simulink model "martins_version_wconv"  (R2023b)
settings: Solver=VariableStepAuto  StartTime=0.0  StopTime=Tend  RelTol=1e-3
undefined symbols (not defined in the file): C_dc, c_f, C_hv_km, Cagg, DiscIntNeverNeededParam, H_vsm, Ibase_hv, Ibase_lv, Ibase_mv, k_AD, k_d_vsm, k_decouple, k_ffv, k_ic, k_idc, k_mod, k_p_p_vsm, k_p_q_vsm, k_pc, k_pdc, k_vc, KG_LL, ki, KI_LL, ki_q, kp, KP_LL, kslope_VSC, L_comp, l_f, l_f_si1, l_grid, L_hv_km, l_t_ehvhv, l_t_hvmv, l_t_mvlv, L_Virt, Lagg, Lbase1v, length_export, omega_nom, P_aero_0, phase_shift_test_state, phase_shifts, pie_export, r_f, r_f_si1, r_grid, R_hv_km, r_t_ehvhv, r_t_hvmv, r_t_mvlv, R_Virt, Ragg, rocof_slope, Rocof_test_state, Sbase1, Tchange_gfm_ref, Tdelay, Trocof_end ... (+13)
libraries: slpidlib x11, spsFirstOrderFilterLib x3, cstblocks x1, simulink x1, spsSampleandHoldLib x1, spspowerguiLib x1
(part 2 of 3)

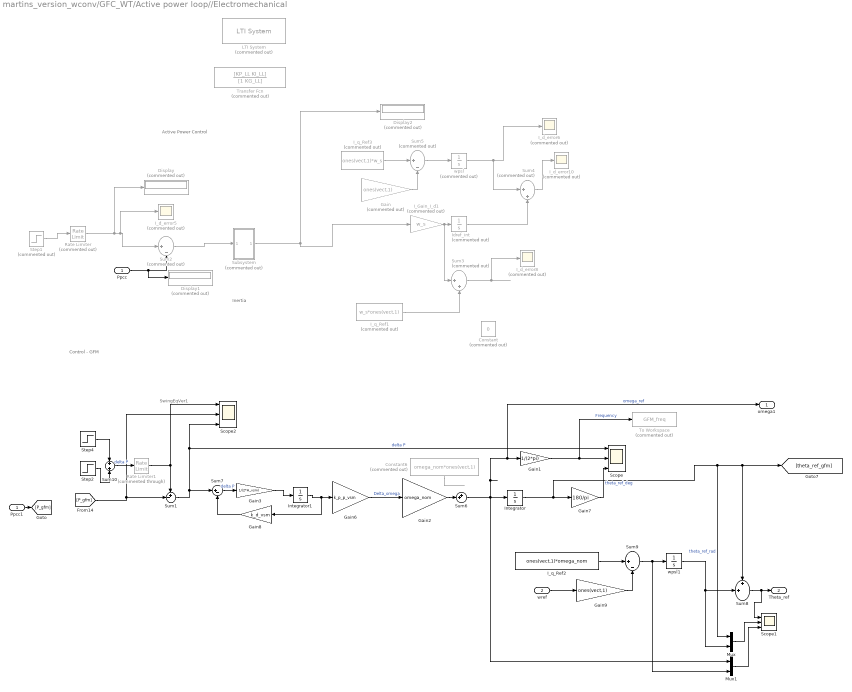
== system martins_version_wconv/GFC_WT/Active power loop//Electromechanical ==
  note: SwingEqVer1
  note: Active Power Control
  note: Inertia
  note: Control - GFM
  Ppcc : Inport  PortDimensions=vect
  wref : Inport  Port=2
  Constant : Constant  Commented=on  Value=0
  Constant6 : Constant  Commented=on  Value=omega_nom*ones(vect,1)
  Display : Display  Commented=on
  Display1 : Display  Commented=on
  Display2 : Display  Commented=on
  Gain : Gain  Commented=on  Gain=ones(vect,1)
  Gain1 : Gain  Gain=1/(2*pi)
  Gain2 : Gain  Gain=omega_nom
  Gain3 : Gain  Gain=1/(2*H_vsm)
  Gain6 : Gain  Gain=k_p_p_vsm
  Gain7 : Gain  Gain=180/pi
  Gain8 : Gain  Gain=k_d_vsm
  Gain9 : Gain  Gain=ones(vect,1)
  I_Gain_I_d1 : Gain  Commented=on  Gain=w_s
  I_d_error{5..6,8,10} (4 alike) : Scope  Commented=on
  I_q_Ref1 : Constant  Commented=on  Value=w_s*ones(vect,1)  SampleTime=-1
  I_q_Ref2 : Constant  Value=ones(vect,1)*omega_nom  SampleTime=-1
  I_q_Ref3 : Constant  Commented=on  Value=ones(vect,1)*w_s  SampleTime=-1
  "Idref_int " : Integrator  Commented=on  UpperSaturationLimit=300  LowerSaturationLimit=-100
  Integrator : Integrator  WrappedStateUpperValue=2*pi  WrappedStateLowerValue=0
  Integrator1 : Integrator
  LTI System : cstblocks/LTI System  Commented=on  sys=sys_mech  IC=[]  PadeOrder=0
  Mux : Mux  Inputs=2
  Mux1 : Mux  Inputs=2
  Ppcc1 : InportShadow  PortDimensions=vect
  Rate Limiter : RateLimiter  Commented=on  RisingSlewLimit=0.5  FallingSlewLimit=-0.5  SampleTimeMode=inherited
  Rate Limiter1 : RateLimiter  Commented=through  RisingSlewLimit=0.5  FallingSlewLimit=-0.5  SampleTimeMode=inherited
  Scope : Scope  NumInputPorts=3
  Scope1 : Scope  NumInputPorts=3
  Scope2 : Scope  NumInputPorts=3
  Step1 : Step  Commented=on  Time=2  Before=ones(vect,1)*0  After=ones(vect,1)*0.9  SampleTime=0
  Step2 : Step  Time=20  Before=0.0*ones(vect,1)  After=1*ones(vect,1)  SampleTime=Ts_power
  Step4 : Step  Time=8  Before=0.0*ones(vect,1)  After=P_aero_0*ones(vect,1)  SampleTime=Ts_power
  Subsystem : Subsystem  Commented=on
  Sum1 : Sum  Inputs=+-|
  Sum10 : Sum
  Sum2 : Sum  Commented=on  Inputs=|+-
  Sum3 : Sum  Commented=on  Inputs=|++
  Sum4 : Sum  Commented=on  Inputs=|++
  Sum5 : Sum  Commented=on  Inputs=|+-
  Sum6 : Sum  Inputs=++|
  Sum7 : Sum  Inputs=|+-
  Sum8 : Sum  Inputs=++|
  Sum9 : Sum  Inputs=|+-
  To Workspace : ToWorkspace  Commented=on  VariableName=GFM_freq  SaveFormat=Structure With Time  SampleTime=-1
  Transfer Fcn : TransferFcn  Commented=on  Numerator=[KP_LL KI_LL]  Denominator=[1 KG_LL]
  wpsl : Integrator  Commented=on  UpperSaturationLimit=300  LowerSaturationLimit=-100
  wpsl1 : Integrator  UpperSaturationLimit=300  LowerSaturationLimit=-100
  omega1 : Outport
  Theta_ref : Outport  Port=2
  wires:
  Ppcc/1 -> Sum2/2, Display1/1
  Subsystem/1(Out1) -> I_Gain_I_d1/1, Display2/1
  Sum4/1 -> I_d_error10/1
  I_Gain_I_d1/1 -> "Idref_int "/1, Sum3/1
  I_q_Ref3/1 -> Sum5/1
  ? -> Gain/1
  Sum5/1 -> wpsl/1
  wpsl/1 -> I_d_error6/1, Sum4/1
  I_q_Ref1/1 -> Sum3/2
  Sum3/1 -> I_d_error8/1
  "Idref_int "/1 -> Sum4/2
  Rate Limiter/1 -> I_d_error5/1, Sum2/1, Display/1
  Sum2/1 -> Subsystem/1(In1)
  Step1/1 -> Rate Limiter/1
  Gain/1 -> Sum5/2
  Step4/1 -> Sum10/1
  Ppcc1/1 -> [P_gfm]
  Gain1/1 -> To Workspace/1, Scope/2  "Frequency"
  Gain2/1 -> Sum6/2
  Constant6/1 -> ?
  Rate Limiter1/1 -> Scope2/1, Sum1/1
  Gain7/1 -> Scope/3  "theta_ref_deg"
  Gain6/1 -> Gain2/1  "Delta_omega"
  Sum6/1 -> Mux1/1, omega1/1, Gain1/1, Integrator/1  "omega_ref"
  Integrator/1 -> Mux/1, Sum8/1, [theta_ref_gfm], Gain7/1  "theta_ref_rad"
  Sum1/1 -> Scope/1, Scope2/3, Sum7/1  "delta P"
  Gain3/1 -> Integrator1/1
  Sum7/1 -> Gain3/1  "delta P"
  Gain8/1 -> Sum7/2
  Integrator1/1 -> Gain6/1, Gain8/1
  wref/1 -> Gain9/1
  wpsl1/1 -> Mux/2, Sum8/2
  I_q_Ref2/1 -> Sum9/1
  Gain9/1 -> Sum9/2
  Sum9/1 -> Mux1/2, wpsl1/1
  Sum8/1 -> Scope1/1, Theta_ref/1
  Mux/1 -> Scope1/2
  Mux1/1 -> Scope1/3
  [P_gfm] -> Sum1/2, Scope2/2
  Sum10/1 -> Rate Limiter1/1  "delta P"
  Step2/1 -> Sum10/2

== system martins_version_wconv/GFC_WT/Current Limit Logic1 ==
  note: Circular Current limiter
  I_ref_unsat : Inport
  Abs1 : Abs
  Constant3 : Constant
  Constant4 : Constant  Value=1.2
  Demux6 : Demux  Outputs=2
  Demux7 : Demux  Outputs=[vect vect]
  Display3 : Display
  Divide : Product  Inputs=*/
  Divide1 : Product  Inputs=*/
  First-Order Filter1 : spsFirstOrderFilterLib/First-Order Filter  FilterType=Lowpass  Tc=0.002  Ts=0  Initialize=on  Vac_Init=[0, 0, 60]  Vdc_Init=0  PlotResponse=off  FreqRange="[0,  200,  1]"
  GreaterThan1 : RelationalOperator  Operator=>  OutDataTypeStr=boolean  RndMeth=Simplest  InputSameDT=off
  I_d_error2 : Scope  Commented=on
  I_d_error3 : Scope  Commented=on
  I_d_error5 : Scope  Commented=on
  Kip12 : Gain
  Kip13 : Gain  Gain=1/1.2
  Mux6 : Mux  Inputs=[vect vect]
  Real-Imag to Complex1 : RealImagToComplex
  Switch1 : Switch  Threshold=1  SaturateOnIntegerOverflow=off  InputSameDT=off
  Unit Delay2 : UnitDelay  InitialCondition=1  SampleTime=-1  HasFrameUpgradeWarning=on
  Vmd2 : Display
  I_ref_sat : Outport
  wires:
  Mux6/1 -> I_ref_sat/1
  Divide1/1 -> Mux6/2
  Demux6/2 -> Real-Imag to Complex1/2
  Abs1/1 -> Kip13/1, I_d_error2/1, GreaterThan1/1
  Unit Delay2/1 -> Divide1/2, Divide/2
  Real-Imag to Complex1/1 -> Abs1/1
  Demux7/2 -> Divide1/1
  GreaterThan1/1 -> Switch1/2
  Demux6/1 -> Real-Imag to Complex1/1
  I_ref_unsat/1 -> Demux7/1, I_d_error5/1, Vmd2/1, First-Order Filter1/1
  Demux7/1 -> Divide/1
  Constant3/1 -> Switch1/3
  Kip13/1 -> Switch1/1
  Constant4/1 -> GreaterThan1/2
  Switch1/1 -> Kip12/1, I_d_error3/1
  Divide/1 -> Mux6/1
  Kip12/1 -> Display3/1, Unit Delay2/1
  First-Order Filter1/1 -> Demux6/1

== system martins_version_wconv/GFC_WT/CurrentControl ==
  note: Analytical tuning
  note: manual tuning
  ref : Inport
  meas : Inport  Port=2
  V grid meas : Inport  Port=3
  Constant : Constant
  Demux : Demux  Outputs=[vect vect]
  Demux1 : Demux  Outputs=[vect vect]
  Demux2 : Demux  Outputs=[vect vect]
  Divide1 : Product  Inputs=**
  Divide2 : Product  Inputs=**
  Gain4 : Gain  Gain=l_f
  Gain5 : Gain  Gain=l_f
  Mux : Mux  Inputs=[vect vect]
  Mux1 : Mux  Inputs=3
  Mux2 : Mux  Inputs=3
  PID Controller : slpidlib/PID Controller  Controller=PI  Form=Ideal  TimeDomain=Continuous-time  UseExternalTs=off  SampleTime=-1  IntegratorMethod=Forward Euler  FilterMethod=Forward Euler  ControllerParametersSource=internal  P=kp  I=ki  UseKiTs=off  D=0  N=100  UseFilter=on  TunerSelectOption=Transfer Function Based (PID Tuner App)  InitialConditionSource=internal  InitialConditionForIntegrator=0  InitialConditionForFilter=0  DifferentiatorICPrevScaledInput=0  ExternalReset=none  TrackingMode=off  Kt=1  LimitOutput=off  SatLimitsSource=internal  UpperSaturationLimit=inf  LowerSaturationLimit=-inf  LinearizeAsGain=on  AntiWindupMode=none  Kb=1  LimitIntegrator=off  UpperIntegratorSaturationLimit=inf  LowerIntegratorSaturationLimit=-inf  POutMin=[]  POutMax=[]  IOutMin=[]  IOutMax=[]  DOutMin=[]  DOutMax=[]  NOutMin=[]  NOutMax=[]  SumOutMin=[]  SumOutMax=[]  SaturationOutMin=[]  SaturationOutMax=[]  PParamMin=[]  PParamMax=[]  IParamMin=[]  IParamMax=[]  DParamMin=[]  DParamMax=[]  NParamMin=[]  NParamMax=[]  KbParamMin=[]  KbParamMax=[]  KtParamMin=[]  KtParamMax=[]  KbOutMin=[]  KbOutMax=[]  KtOutMin=[]  KtOutMax=[]  IntegratorOutMin=[]  IntegratorOutMax=[]  FilterOutMin=[]  FilterOutMax=[]  SumI1OutMin=[]  SumI1OutMax=[]  SumI2OutMin=[]  SumI2OutMax=[]  SumI3OutMin=[]  SumI3OutMax=[]  SumI4OutMin=[]  SumI4OutMax=[]  SumDOutMin=[]  SumDOutMax=[]  DifferentiatorOutMin=[]  DifferentiatorOutMax=[]  FilterDiffOutCoefMin=[]  FilterDiffOutCoefMax=[]  ReciprocalOutMin=[]  ReciprocalOutMax=[]  SumDenOutMin=[]  SumDenOutMax=[]  SumNumOutMin=[]  SumNumOutMax=[]  DivideOutMin=[]  DivideOutMax=[]  UdiffTsProdOutMin=[]  UdiffTsProdOutMax=[]  NTsProdOutMin=[]  NTsProdOutMax=[]  UintegralTsProdOutMin=[]  UintegralTsProdOutMax=[]  UngainTsProdOutMin=[]  UngainTsProdOutMax=[]  ClampingZeroOutDataTypeStr=Inherit: Inherit via back propagation  ClampingZeroOutMin=[]  ClampingZeroOutMax=[]  FilterDenConstantOutDataTypeStr=Inherit: Inherit via back propagation  FilterDenConstantOutMin=[]  FilterDenConstantOutMax=[]  PCopyOutDataTypeStr=Inherit: Inherit via back propagation  PCopyOutMin=[]  PCopyOutMax=[]  NCopyOutDataTypeStr=Inherit: Inherit via back propagation  NCopyOutMin=[]  NCopyOutMax=[]  IntegratorContinuousStateAttributes=''  IntegratorStateMustResolveToSignalObject=off  IntegratorRTWStateStorageClass=Auto  FilterContinuousStateAttributes=''  FilterStateMustResolveToSignalObject=off  FilterRTWStateStorageClass=Auto  ParallelPVariant=Passthrough  IdealPVariant=InternalParameters  IVariant=InternalParameters  DVariant=Disabled  IntegratorVariant=Continuous  SatVariant=Disabled  AWVariant=Passthrough  PCopyVariant=Disabled  TRVariant=Disabled  FdbkBlocksVariant=Forward  IdealPFdbkVariant=Disabled  SatFdbkVariant=Disabled  DerivativeFilterVariant=Disabled  NVariant=Disabled  NCopyVariant=Disabled_SignalSpec  FilterICVariant=Disabled  IntegratorICVariant=InternalICs  ExternalResetVariant=Disabled  TRSumVariant=Passthrough  SumFdbkVariant=Disabled  SumVariant=Sum_PI  TsampFilterVariant=InternalTs  TsampNgainVariant=Passthrough  TsampIntegralVariant=Disabled_SignalSpec  ExternalSaturationOutDataTypeStr=Inherit: Same as second input
  PID Controller1 : slpidlib/PID Controller  Controller=PI  Form=Ideal  TimeDomain=Continuous-time  UseExternalTs=off  SampleTime=-1  IntegratorMethod=Forward Euler  FilterMethod=Forward Euler  ControllerParametersSource=internal  P=kp  I=ki  UseKiTs=off  D=0  N=100  UseFilter=on  TunerSelectOption=Transfer Function Based (PID Tuner App)  InitialConditionSource=internal  InitialConditionForIntegrator=1  InitialConditionForFilter=0  DifferentiatorICPrevScaledInput=0  ExternalReset=none  TrackingMode=off  Kt=1  LimitOutput=off  SatLimitsSource=internal  UpperSaturationLimit=inf  LowerSaturationLimit=-inf  LinearizeAsGain=on  AntiWindupMode=none  Kb=1  LimitIntegrator=off  UpperIntegratorSaturationLimit=inf  LowerIntegratorSaturationLimit=-inf  POutMin=[]  POutMax=[]  IOutMin=[]  IOutMax=[]  DOutMin=[]  DOutMax=[]  NOutMin=[]  NOutMax=[]  SumOutMin=[]  SumOutMax=[]  SaturationOutMin=[]  SaturationOutMax=[]  PParamMin=[]  PParamMax=[]  IParamMin=[]  IParamMax=[]  DParamMin=[]  DParamMax=[]  NParamMin=[]  NParamMax=[]  KbParamMin=[]  KbParamMax=[]  KtParamMin=[]  KtParamMax=[]  KbOutMin=[]  KbOutMax=[]  KtOutMin=[]  KtOutMax=[]  IntegratorOutMin=[]  IntegratorOutMax=[]  FilterOutMin=[]  FilterOutMax=[]  SumI1OutMin=[]  SumI1OutMax=[]  SumI2OutMin=[]  SumI2OutMax=[]  SumI3OutMin=[]  SumI3OutMax=[]  SumI4OutMin=[]  SumI4OutMax=[]  SumDOutMin=[]  SumDOutMax=[]  DifferentiatorOutMin=[]  DifferentiatorOutMax=[]  FilterDiffOutCoefMin=[]  FilterDiffOutCoefMax=[]  ReciprocalOutMin=[]  ReciprocalOutMax=[]  SumDenOutMin=[]  SumDenOutMax=[]  SumNumOutMin=[]  SumNumOutMax=[]  DivideOutMin=[]  DivideOutMax=[]  UdiffTsProdOutMin=[]  UdiffTsProdOutMax=[]  NTsProdOutMin=[]  NTsProdOutMax=[]  UintegralTsProdOutMin=[]  UintegralTsProdOutMax=[]  UngainTsProdOutMin=[]  UngainTsProdOutMax=[]  ClampingZeroOutDataTypeStr=Inherit: Inherit via back propagation  ClampingZeroOutMin=[]  ClampingZeroOutMax=[]  FilterDenConstantOutDataTypeStr=Inherit: Inherit via back propagation  FilterDenConstantOutMin=[]  FilterDenConstantOutMax=[]  PCopyOutDataTypeStr=Inherit: Inherit via back propagation  PCopyOutMin=[]  PCopyOutMax=[]  NCopyOutDataTypeStr=Inherit: Inherit via back propagation  NCopyOutMin=[]  NCopyOutMax=[]  IntegratorContinuousStateAttributes=''  IntegratorStateMustResolveToSignalObject=off  IntegratorRTWStateStorageClass=Auto  FilterContinuousStateAttributes=''  FilterStateMustResolveToSignalObject=off  FilterRTWStateStorageClass=Auto  ParallelPVariant=Passthrough  IdealPVariant=InternalParameters  IVariant=InternalParameters  DVariant=Disabled  IntegratorVariant=Continuous  SatVariant=Disabled  AWVariant=Passthrough  PCopyVariant=Disabled  TRVariant=Disabled  FdbkBlocksVariant=Forward  IdealPFdbkVariant=Disabled  SatFdbkVariant=Disabled  DerivativeFilterVariant=Disabled  NVariant=Disabled  NCopyVariant=Disabled_SignalSpec  FilterICVariant=Disabled  IntegratorICVariant=InternalICs  ExternalResetVariant=Disabled  TRSumVariant=Passthrough  SumFdbkVariant=Disabled  SumVariant=Sum_PI  TsampFilterVariant=InternalTs  TsampNgainVariant=Passthrough  TsampIntegralVariant=Disabled_SignalSpec  ExternalSaturationOutDataTypeStr=Inherit: Same as second input
  PID Controller2 : slpidlib/PID Controller  Controller=PI  Form=Ideal  TimeDomain=Continuous-time  UseExternalTs=off  SampleTime=-1  IntegratorMethod=Forward Euler  FilterMethod=Forward Euler  ControllerParametersSource=internal  P=0.06  I=1/0.0013  UseKiTs=off  D=0  N=100  UseFilter=on  TunerSelectOption=Transfer Function Based (PID Tuner App)  InitialConditionSource=internal  InitialConditionForIntegrator=1  InitialConditionForFilter=0  DifferentiatorICPrevScaledInput=0  ExternalReset=none  TrackingMode=off  Kt=1  LimitOutput=off  SatLimitsSource=internal  UpperSaturationLimit=inf  LowerSaturationLimit=-inf  LinearizeAsGain=on  AntiWindupMode=none  Kb=1  LimitIntegrator=off  UpperIntegratorSaturationLimit=inf  LowerIntegratorSaturationLimit=-inf  POutMin=[]  POutMax=[]  IOutMin=[]  IOutMax=[]  DOutMin=[]  DOutMax=[]  NOutMin=[]  NOutMax=[]  SumOutMin=[]  SumOutMax=[]  SaturationOutMin=[]  SaturationOutMax=[]  PParamMin=[]  PParamMax=[]  IParamMin=[]  IParamMax=[]  DParamMin=[]  DParamMax=[]  NParamMin=[]  NParamMax=[]  KbParamMin=[]  KbParamMax=[]  KtParamMin=[]  KtParamMax=[]  KbOutMin=[]  KbOutMax=[]  KtOutMin=[]  KtOutMax=[]  IntegratorOutMin=[]  IntegratorOutMax=[]  FilterOutMin=[]  FilterOutMax=[]  SumI1OutMin=[]  SumI1OutMax=[]  SumI2OutMin=[]  SumI2OutMax=[]  SumI3OutMin=[]  SumI3OutMax=[]  SumI4OutMin=[]  SumI4OutMax=[]  SumDOutMin=[]  SumDOutMax=[]  DifferentiatorOutMin=[]  DifferentiatorOutMax=[]  FilterDiffOutCoefMin=[]  FilterDiffOutCoefMax=[]  ReciprocalOutMin=[]  ReciprocalOutMax=[]  SumDenOutMin=[]  SumDenOutMax=[]  SumNumOutMin=[]  SumNumOutMax=[]  DivideOutMin=[]  DivideOutMax=[]  UdiffTsProdOutMin=[]  UdiffTsProdOutMax=[]  NTsProdOutMin=[]  NTsProdOutMax=[]  UintegralTsProdOutMin=[]  UintegralTsProdOutMax=[]  UngainTsProdOutMin=[]  UngainTsProdOutMax=[]  ClampingZeroOutDataTypeStr=Inherit: Inherit via back propagation  ClampingZeroOutMin=[]  ClampingZeroOutMax=[]  FilterDenConstantOutDataTypeStr=Inherit: Inherit via back propagation  FilterDenConstantOutMin=[]  FilterDenConstantOutMax=[]  PCopyOutDataTypeStr=Inherit: Inherit via back propagation  PCopyOutMin=[]  PCopyOutMax=[]  NCopyOutDataTypeStr=Inherit: Inherit via back propagation  NCopyOutMin=[]  NCopyOutMax=[]  IntegratorContinuousStateAttributes=''  IntegratorStateMustResolveToSignalObject=off  IntegratorRTWStateStorageClass=Auto  FilterContinuousStateAttributes=''  FilterStateMustResolveToSignalObject=off  FilterRTWStateStorageClass=Auto  ParallelPVariant=Passthrough  IdealPVariant=InternalParameters  IVariant=InternalParameters  DVariant=Disabled  IntegratorVariant=Continuous  SatVariant=Disabled  AWVariant=Passthrough  PCopyVariant=Disabled  TRVariant=Disabled  FdbkBlocksVariant=Forward  IdealPFdbkVariant=Disabled  SatFdbkVariant=Disabled  DerivativeFilterVariant=Disabled  NVariant=Disabled  NCopyVariant=Disabled_SignalSpec  FilterICVariant=Disabled  IntegratorICVariant=InternalICs  ExternalResetVariant=Disabled  TRSumVariant=Passthrough  SumFdbkVariant=Disabled  SumVariant=Sum_PI  TsampFilterVariant=InternalTs  TsampNgainVariant=Passthrough  TsampIntegralVariant=Disabled_SignalSpec  ExternalSaturationOutDataTypeStr=Inherit: Same as second input
  PID Controller3 : slpidlib/PID Controller  Controller=PI  Form=Ideal  TimeDomain=Continuous-time  UseExternalTs=off  SampleTime=-1  IntegratorMethod=Forward Euler  FilterMethod=Forward Euler  ControllerParametersSource=internal  P=0.06  I=1/0.0013  UseKiTs=off  D=0  N=100  UseFilter=on  TunerSelectOption=Transfer Function Based (PID Tuner App)  InitialConditionSource=internal  InitialConditionForIntegrator=0  InitialConditionForFilter=0  DifferentiatorICPrevScaledInput=0  ExternalReset=none  TrackingMode=off  Kt=1  LimitOutput=off  SatLimitsSource=internal  UpperSaturationLimit=inf  LowerSaturationLimit=-inf  LinearizeAsGain=on  AntiWindupMode=none  Kb=1  LimitIntegrator=off  UpperIntegratorSaturationLimit=inf  LowerIntegratorSaturationLimit=-inf  POutMin=[]  POutMax=[]  IOutMin=[]  IOutMax=[]  DOutMin=[]  DOutMax=[]  NOutMin=[]  NOutMax=[]  SumOutMin=[]  SumOutMax=[]  SaturationOutMin=[]  SaturationOutMax=[]  PParamMin=[]  PParamMax=[]  IParamMin=[]  IParamMax=[]  DParamMin=[]  DParamMax=[]  NParamMin=[]  NParamMax=[]  KbParamMin=[]  KbParamMax=[]  KtParamMin=[]  KtParamMax=[]  KbOutMin=[]  KbOutMax=[]  KtOutMin=[]  KtOutMax=[]  IntegratorOutMin=[]  IntegratorOutMax=[]  FilterOutMin=[]  FilterOutMax=[]  SumI1OutMin=[]  SumI1OutMax=[]  SumI2OutMin=[]  SumI2OutMax=[]  SumI3OutMin=[]  SumI3OutMax=[]  SumI4OutMin=[]  SumI4OutMax=[]  SumDOutMin=[]  SumDOutMax=[]  DifferentiatorOutMin=[]  DifferentiatorOutMax=[]  FilterDiffOutCoefMin=[]  FilterDiffOutCoefMax=[]  ReciprocalOutMin=[]  ReciprocalOutMax=[]  SumDenOutMin=[]  SumDenOutMax=[]  SumNumOutMin=[]  SumNumOutMax=[]  DivideOutMin=[]  DivideOutMax=[]  UdiffTsProdOutMin=[]  UdiffTsProdOutMax=[]  NTsProdOutMin=[]  NTsProdOutMax=[]  UintegralTsProdOutMin=[]  UintegralTsProdOutMax=[]  UngainTsProdOutMin=[]  UngainTsProdOutMax=[]  ClampingZeroOutDataTypeStr=Inherit: Inherit via back propagation  ClampingZeroOutMin=[]  ClampingZeroOutMax=[]  FilterDenConstantOutDataTypeStr=Inherit: Inherit via back propagation  FilterDenConstantOutMin=[]  FilterDenConstantOutMax=[]  PCopyOutDataTypeStr=Inherit: Inherit via back propagation  PCopyOutMin=[]  PCopyOutMax=[]  NCopyOutDataTypeStr=Inherit: Inherit via back propagation  NCopyOutMin=[]  NCopyOutMax=[]  IntegratorContinuousStateAttributes=''  IntegratorStateMustResolveToSignalObject=off  IntegratorRTWStateStorageClass=Auto  FilterContinuousStateAttributes=''  FilterStateMustResolveToSignalObject=off  FilterRTWStateStorageClass=Auto  ParallelPVariant=Passthrough  IdealPVariant=InternalParameters  IVariant=InternalParameters  DVariant=Disabled  IntegratorVariant=Continuous  SatVariant=Disabled  AWVariant=Passthrough  PCopyVariant=Disabled  TRVariant=Disabled  FdbkBlocksVariant=Forward  IdealPFdbkVariant=Disabled  SatFdbkVariant=Disabled  DerivativeFilterVariant=Disabled  NVariant=Disabled  NCopyVariant=Disabled_SignalSpec  FilterICVariant=Disabled  IntegratorICVariant=InternalICs  ExternalResetVariant=Disabled  TRSumVariant=Passthrough  SumFdbkVariant=Disabled  SumVariant=Sum_PI  TsampFilterVariant=InternalTs  TsampNgainVariant=Passthrough  TsampIntegralVariant=Disabled_SignalSpec  ExternalSaturationOutDataTypeStr=Inherit: Same as second input
  Step1 : Step  Before=1  SampleTime=0
  Step2 : Step  Before=1  SampleTime=0
  Sum1 : Sum  Inputs=|+-
  Sum2 : Sum  Inputs=+-|
  Sum4 : Sum  Inputs=++-
  Sum5 : Sum  Inputs=+++
  Transfer Fcn2 : TransferFcn  Denominator=[0.005 1]
  Transfer Fcn3 : TransferFcn  Denominator=[0.005 1]
  d-axis-control : Scope  NumInputPorts=3
  q-axis control : Scope  NumInputPorts=3
  Out1 : Outport
  wires:
  Step2/1 -> Divide1/2
  Sum2/1 -> q-axis control/1, Divide1/1
  Mux2/1 -> q-axis control/2
  PID Controller2/1 -> Sum4/2, Mux1/2
  Step1/1 -> Divide2/2
  Divide2/1 -> PID Controller2/1
  Divide1/1 -> PID Controller3/1
  Transfer Fcn3/1 -> Mux2/1, Sum5/3
  ref/1 -> Demux/1
  Gain4/1 -> Mux2/3, Sum5/1
  Transfer Fcn2/1 -> Mux1/1, Sum4/1
  Gain5/1 -> Mux1/3, Sum4/3
  V grid meas/1 -> Demux2/1
  Mux1/1 -> d-axis-control/2
  Sum4/1 -> d-axis-control/3, Mux/1
  Demux2/2 -> Transfer Fcn3/1
  Sum5/1 -> q-axis control/3, Mux/2
  PID Controller3/1 -> Mux2/2, Sum5/2
  meas/1 -> Demux1/1
  Demux/1 -> Sum1/1
  Mux/1 -> Out1/1
  Demux/2 -> Sum2/1
  Demux1/1 -> Gain4/1, Sum1/2
  Demux1/2 -> Gain5/1, Sum2/2
  Sum1/1 -> Divide2/1, d-axis-control/1
  Demux2/1 -> Transfer Fcn2/1

== system martins_version_wconv/GFC_WT/DC-link voltage controller ==
  ref : Inport
  meas : Inport  Port=2
  DC init : Subsystem
  Gain : Gain
  Gain1 : Gain
  Hit Crossing : HitCross
  Mux : Mux  Inputs=2
  PID Controller : slpidlib/PID Controller  Controller=PI  Form=Parallel  TimeDomain=Continuous-time  UseExternalTs=off  SampleTime=-1  IntegratorMethod=Forward Euler  FilterMethod=Forward Euler  ControllerParametersSource=internal  P=2  I=5  UseKiTs=off  D=0.0506  N=100  UseFilter=on  TunerSelectOption=Transfer Function Based (PID Tuner App)  InitialConditionSource=internal  InitialConditionForIntegrator=0  InitialConditionForFilter=0  DifferentiatorICPrevScaledInput=0  ExternalReset=none  TrackingMode=off  Kt=1  LimitOutput=off  SatLimitsSource=internal  UpperSaturationLimit=0.5  LowerSaturationLimit=-0.5  LinearizeAsGain=on  AntiWindupMode=clamping  Kb=1  LimitIntegrator=off  UpperIntegratorSaturationLimit=0.5  LowerIntegratorSaturationLimit=-0.5  POutMin=[]  POutMax=[]  IOutMin=[]  IOutMax=[]  DOutMin=[]  DOutMax=[]  NOutMin=[]  NOutMax=[]  SumOutMin=[]  SumOutMax=[]  SaturationOutMin=[]  SaturationOutMax=[]  PParamMin=[]  PParamMax=[]  IParamMin=[]  IParamMax=[]  DParamMin=[]  DParamMax=[]  NParamMin=[]  NParamMax=[]  KbParamMin=[]  KbParamMax=[]  KtParamMin=[]  KtParamMax=[]  KbOutMin=[]  KbOutMax=[]  KtOutMin=[]  KtOutMax=[]  IntegratorOutMin=[]  IntegratorOutMax=[]  FilterOutMin=[]  FilterOutMax=[]  SumI1OutMin=[]  SumI1OutMax=[]  SumI2OutMin=[]  SumI2OutMax=[]  SumI3OutMin=[]  SumI3OutMax=[]  SumI4OutMin=[]  SumI4OutMax=[]  SumDOutMin=[]  SumDOutMax=[]  DifferentiatorOutMin=[]  DifferentiatorOutMax=[]  FilterDiffOutCoefMin=[]  FilterDiffOutCoefMax=[]  ReciprocalOutMin=[]  ReciprocalOutMax=[]  SumDenOutMin=[]  SumDenOutMax=[]  SumNumOutMin=[]  SumNumOutMax=[]  DivideOutMin=[]  DivideOutMax=[]  UdiffTsProdOutMin=[]  UdiffTsProdOutMax=[]  NTsProdOutMin=[]  NTsProdOutMax=[]  UintegralTsProdOutMin=[]  UintegralTsProdOutMax=[]  UngainTsProdOutMin=[]  UngainTsProdOutMax=[]  ClampingZeroOutDataTypeStr=Inherit: Inherit via back propagation  ClampingZeroOutMin=[]  ClampingZeroOutMax=[]  FilterDenConstantOutDataTypeStr=Inherit: Inherit via back propagation  FilterDenConstantOutMin=[]  FilterDenConstantOutMax=[]  PCopyOutDataTypeStr=Inherit: Inherit via back propagation  PCopyOutMin=[]  PCopyOutMax=[]  NCopyOutDataTypeStr=Inherit: Inherit via back propagation  NCopyOutMin=[]  NCopyOutMax=[]  IntegratorContinuousStateAttributes=''  IntegratorStateMustResolveToSignalObject=off  IntegratorRTWStateStorageClass=Auto  FilterContinuousStateAttributes=''  FilterStateMustResolveToSignalObject=off  FilterRTWStateStorageClass=Auto  ParallelPVariant=InternalParameters  IdealPVariant=Disabled  IVariant=InternalParameters  DVariant=Disabled  IntegratorVariant=Continuous  SatVariant=Disabled  AWVariant=Passthrough  PCopyVariant=Disabled  TRVariant=Disabled  FdbkBlocksVariant=Forward  IdealPFdbkVariant=Disabled  SatFdbkVariant=Disabled  DerivativeFilterVariant=Disabled  NVariant=Disabled  NCopyVariant=Disabled_SignalSpec  FilterICVariant=Disabled  IntegratorICVariant=InternalICs  ExternalResetVariant=Disabled  TRSumVariant=Passthrough  SumFdbkVariant=Disabled  SumVariant=Sum_PI  TsampFilterVariant=InternalTs  TsampNgainVariant=Passthrough  TsampIntegralVariant=Disabled_SignalSpec  ExternalSaturationOutDataTypeStr=Inherit: Same as second input
  Square : Math  Operator=square
  Square1 : Math  Operator=square
  Sum : Sum  Inputs=+-|
  Transfer Fcn : TransferFcn  Numerator=[8]  Denominator=[1 4*0.707 8]
  input : Outport
  error : Outport  Port=2
  out : Outport  Port=3
  Out4 : Outport  Port=4
  wires:
  Mux/1 -> input/1
  PID Controller/1 -> out/1, Gain/1
  Gain/1 -> Out4/1
  Sum/1 -> Hit Crossing/1, error/1, Gain1/1
  meas/1 -> Square/1
  ref/1 -> Square1/1
  Square/1 -> Mux/2, Sum/2
  Square1/1 -> Mux/1, Sum/1
  Gain1/1 -> PID Controller/1
  Transfer Fcn/1 -> ?
  Hit Crossing/1 -> ?

== system martins_version_wconv/GFC_WT/PLL>>grid1 ==
  note: inv ([  cos(wt)   sin(wt)
      |    -sin(wt)    cos(wt)   ])
  note: =
  note: [  al
      |     be  ]
  note: =
  note: [  al
      |     be  ]
  note: [ d
      |    q ]
  note: *
  note: [ d
      |    q ]
  note: [  cos(wt)   -sin(wt)
      |    sin(wt)    cos(wt)   ]
  note: *
  vgdq : Inport
  thetaPLL : Inport  Port=2
  Cos : Trigonometry  Operator=cos
  Demux1 : Demux  Outputs=2
  Display5 : Display
  Mux3 : Mux  Inputs=2
  Product{,1..3} (4 alike) : Product
  Sin : Trigonometry
  Sum : Sum  Inputs=+-
  Sum1 : Sum
  vgDQ : Outport  InitialOutput=[0,0]  VectorParamsAs1DForOutWhenUnconnected=off
  wires:
  vgdq/1 -> Demux1/1
  thetaPLL/1 -> Cos/1, Sin/1
  Sin/1 -> Product3/2, Product1/2
  Demux1/1 -> Product3/1, Product/1
  Cos/1 -> Product2/2, Product/2
  Product/1 -> Sum/1
  Demux1/2 -> Product2/1, Product1/1
  Product1/1 -> Sum/2
  Sum/1 -> Mux3/1
  Product2/1 -> Sum1/1
  Product3/1 -> Sum1/2
  Sum1/1 -> Mux3/2
  Mux3/1 -> Display5/1, vgDQ/1

== system martins_version_wconv/GFC_WT/PQ PCC ==
  note: PQ VSC bus
  IDQ : Inport
  VDQ : Inport  Port=2
  Demux7 : Demux  Outputs=[vect vect]
  Demux8 : Demux  Outputs=[vect vect]
  Product{1,3..5} (4 alike) : Product  InputSameDT=on  SaturateOnIntegerOverflow=on  OutDataTypeStr=Inherit: Same as first input
  Sum : Sum  InputSameDT=on  SaturateOnIntegerOverflow=on  OutDataTypeStr=Inherit: Same as first input
  Sum1 : Sum  Inputs=+-  InputSameDT=on  SaturateOnIntegerOverflow=on  OutDataTypeStr=Inherit: Same as first input
  P : Outport
  Q : Outport  Port=2
  wires:
  Product5/1 -> Sum1/2
  Product1/1 -> Sum1/1
  Demux8/2 -> Product1/1, Product4/1
  Demux7/1 -> Product1/2, Product3/1
  Demux8/1 -> Product5/1, Product3/2
  Product4/1 -> Sum/2
  Demux7/2 -> Product4/2, Product5/2
  Product3/1 -> Sum/1
  VDQ/1 -> Demux8/1
  Sum1/1 -> Q/1
  IDQ/1 -> Demux7/1
  Sum/1 -> P/1

== system martins_version_wconv/GFC_WT/PQ Virtual Bus1 ==
  note: PQ Virtual bus
  IDQ : Inport
  VDQ : Inport  Port=2
  Demux5 : Demux  Outputs=[vect vect]
  Demux6 : Demux  Outputs=[vect vect]
  Product{1,3..5} (4 alike) : Product  InputSameDT=on  SaturateOnIntegerOverflow=on  OutDataTypeStr=Inherit: Same as first input
  Sum : Sum  InputSameDT=on  SaturateOnIntegerOverflow=on  OutDataTypeStr=Inherit: Same as first input
  Sum1 : Sum  Inputs=+-  InputSameDT=on  SaturateOnIntegerOverflow=on  OutDataTypeStr=Inherit: Same as first input
  P : Outport
  Q : Outport  Port=2
  wires:
  Sum/1 -> P/1
  VDQ/1 -> Demux6/1
  IDQ/1 -> Demux5/1
  Sum1/1 -> Q/1
  Product5/1 -> Sum1/2
  Product1/1 -> Sum1/1
  Demux6/2 -> Product4/1, Product1/1
  Demux5/1 -> Product1/2, Product3/1
  Demux6/1 -> Product3/2, Product5/1
  Product4/1 -> Sum/2
  Demux5/2 -> Product5/2, Product4/2
  Product3/1 -> Sum/1

== system martins_version_wconv/GFC_WT/RL filter1 ==
  note: Inverter side inductor
  In1 : Inport
  In2 : Inport  Port=2
  In3 : Inport  Port=3
  In4 : Inport  Port=4
  In5 : Inport  Port=5
  1 : Gain  Gain=r_f*Zbase1v
  2 : Gain  Gain=1/(l_f*Lbase1v)
  3 : Gain  Gain=r_f*Zbase1v
  4 : Gain  Gain=1/(l_f*Lbase1v)
  Id : Scope
  Id_int : Integrator  UpperSaturationLimit=50  LowerSaturationLimit=-1000
  Iq : Scope
  Iq_int : Integrator  UpperSaturationLimit=50  LowerSaturationLimit=-1000
  L value : Constant  Value=l_f*Lbase1v  SampleTime=-1
  Product : Product
  Product1 : Product
  Product2 : Product
  Sum1 : Sum  Inputs=|+---
  Sum8 : Sum  Inputs=|+-+-
  id1 : Display
  Out1 : Outport
  Out2 : Outport  Port=2
  wires:
  In5/1 -> Product/1
  Product/1 -> [wL], id1/1
  L value/1 -> Product/2
  In1/1 -> Sum1/2
  In3/1 -> Sum1/1
  In4/1 -> Sum8/2
  In2/1 -> Sum8/1
  Product2/1 -> Sum8/3
  Iq_int/1 -> Iq/1, Product2/2, 3/1, Out1/1
  4/1 -> Iq_int/1
  Sum8/1 -> 2/1
  2/1 -> Id_int/1
  Sum1/1 -> 4/1
  3/1 -> Sum1/4
  Product1/1 -> Sum1/3
  1/1 -> Sum8/4
  Id_int/1 -> Product1/2, Out2/1, Id/1, 1/1
  [wL] -> Product1/1, Product2/1

== system martins_version_wconv/GFC_WT/Reactive Power //AVR ==
  note: Voltage control
  note: IQref
  Vmag : Inport
  Qmeas : Inport  Port=2
  Constant5 : Constant
  Gain1 : Gain
  Gain3 : Gain  Commented=through  Gain=ki_q
  Gain8 : Gain  Commented=through  Gain=1/Sbase1
  Gain9 : Gain  Gain=k_p_q_vsm
  I_Gain_I_d3 : Gain  Commented=on  Gain=kslope_VSC
  I_d_error{1,3..5} (4 alike) : Scope  Commented=on
  I_q_Ref1 : Constant  Commented=on  Value=ones(vect,1)  SampleTime=-1
  Integrator : Integrator  Commented=on  LimitOutput=on  UpperSaturationLimit=0.2  LowerSaturationLimit=-0.2
  Integrator1 : Integrator  Commented=through
  Kip1 : Gain  Commented=on  Gain=10
  Qmeas1 : InportShadow  Port=2
  Qref1 : Constant  Value=0.0  SampleTime=Ts_power
  Scope : Scope  NumInputPorts=4
  Scope7 : Scope  NumInputPorts=2
  Step : Step  Commented=on  Time=2  Before=1  SampleTime=0
  Step2 : Step  Commented=on  Time=2  After=0  SampleTime=0
  Sum1 : Sum  Commented=on  Inputs=|+-+
  Sum3 : Sum  Inputs=|-+
  Sum4 : Sum  Inputs=|++
  Sum7 : Sum  Inputs=|+-
  Transfer Fcn1 : TransferFcn  Numerator=[ki_q]  Denominator=[1 ki_q]
  V_nominal : Constant  Value=ones(vect,1)
  Delta_V : Outport
  V_ref_d : Outport  Port=2
  wires:
  Kip1/1 -> Integrator/1
  Step/1 -> Sum1/1
  I_Gain_I_d3/1 -> Sum1/3, I_d_error5/1
  Qmeas/1 -> I_Gain_I_d3/1, I_d_error4/1
  Sum1/1 -> Kip1/1
  Integrator/1 -> I_d_error3/1, Delta_V/1
  Vmag/1 -> I_d_error1/1, Sum1/2
  [Q_grid] -> Gain8/1  "Gen Reactive Power"
  Qmeas1/1 -> [Q_grid]
  V_nominal/1 -> Sum4/2
  Gain8/1 -> Sum3/1
  Qref1/1 -> Sum3/2
  Sum4/1 -> V_ref_d/1, Scope7/1, Scope/4  "Vref"
  Sum3/1 -> Transfer Fcn1/1, Sum7/1, Scope7/2, Scope/1  "delta Q"
  Integrator1/1 -> Gain9/1, Scope/2, Gain1/1
  Gain9/1 -> Scope/3, Sum4/1
  Constant5/1 -> ?
  Gain3/1 -> Integrator1/1
  Sum7/1 -> Gain3/1
  Gain1/1 -> ?

== system martins_version_wconv/GFC_WT/Subsystem ==
  In1 : Inport
  In2 : Inport  Port=2
  omega_PLL : Inport  Port=3
  omega_ref : Inport  Port=4
  In4 : Inport  Port=5
  Constant : Constant  Commented=on  Value=Tdelay*w_s
  Current Control : Subsystem  Commented=on
  Current Limit Logic : Subsystem  Commented=through
  Demux4 : Demux  Commented=on  Outputs=2
  First-Order Filter : spsFirstOrderFilterLib/First-Order Filter  Commented=on  FilterType=Lowpass  Tc=0.02  Ts=0  Initialize=on  Vac_Init=[0, 0, 60]  Vdc_Init=0  PlotResponse=off  FreqRange="[0,  200,  1]"
  From1 : From  Commented=on  GotoTag=Idq
  From17 : From  Commented=on  GotoTag=vQ
  From18 : From  Commented=on  GotoTag=vD
  From2 : From  Commented=on  GotoTag=thetaPLL
  From4 : From  Commented=on  GotoTag=vdq
  From5 : From  Commented=on  GotoTag=Iodq
  Goto3 : Goto  Commented=on  GotoTag=IQ
  Goto4 : Goto  Commented=on  GotoTag=ID
  I_d_error4 : Scope  Commented=on
  Kip6 : Gain  Commented=on  Gain=Vbase_lv
  Kip9 : Gain  Commented=through  Gain=1/Vbase_lv_pk
  PLL>>grid2 : Subsystem  Commented=on  AncestorBlock=powerlib_meascontrol/Transformations/Alpha-Beta-Zero to dq0/Subsystem - pi//2 delay
  Product : Product  Commented=on  Inputs=**  InputSameDT=on  SaturateOnIntegerOverflow=on  OutDataTypeStr=Inherit: Same as first input
  RL filter : Subsystem  Commented=on
      settings: PortSchema="{\"entries\":[{\"content\":{\"sides\":[{\"content\":{\"connectorIds\":[\"In1\",\"In2\",\"In3\",\"In4\"]},\"type\":\"ConnectorPlacement.EquallySpacedRectSide\",\"uuid\":\"57ad71d1-5664-4b35-a20c-d71f7e1cdc47\"},{\"content\":{\"connectorIds\":[\"Out1\",\"Out2\"],\"side\":\"RIGHT\"},\"type\":\"ConnectorPlacement.EquallySpacedRectSide\",\"uuid\":\"8101605d-eedb-4c26-847d-0cc0ce629d60\"},{\"content\":{\"connectorIds\":[],\"side\":\"TOP\"},\"type\":\"ConnectorPlacement.EquallySpacedRectSide\",\"uuid\":\"2627b00b-24a5-469a-be2d-9c3c8a1d2080\"},{\"content\":{\"connectorIds\":[\"In5\"],\"side\":\"BOTTOM\"},\"type\":\"ConnectorPlacement.EquallySpacedRectSide\",\"uuid\":\"fe553db7-7727-4a02-b1e7-5aedfb7840ee\"}]},\"type\":\"ConnectorPlacement.EquallySpacedConnector\",\"uuid\":\"f40200c8-ad5b-428c-8a4e-7641595b86c4\"}],\"packageUris\":[\"http://schema.mathworks.com/mf0/Connector/19700101\"],\"version\":\"1.0\"}"
  Step : Step  Commented=on  Before=1  After=0  SampleTime=0
  Sum1 : Sum  Commented=on  Inputs=|+-
  Sum2 : Sum  Commented=on  Inputs=|+-
  Switch : Switch  Commented=on  Criteria=u2 > Threshold  SaturateOnIntegerOverflow=off  InputSameDT=off
  Transport Delay : TransportDelay  Commented=on  DelayTime=Tdelay/2
  Transport Delay1 : TransportDelay  Commented=on  DelayTime=Tdelay/2
  Vdc value for converter AC output of 1 pu for m=1 : Constant  Commented=on  Value=1/k_mod
  Virtual Admittance1 : Subsystem  Commented=on
  Vmd13 : Display  Commented=on
  wires:
  Demux4/2 -> Transport Delay1/1
  Transport Delay/1 -> RL filter/2(In2)
  RL filter/2(Out2) -> Goto4/1
  Demux4/1 -> Transport Delay/1
  RL filter/1(Out1) -> Goto3/1
  Vdc value for converter AC output of 1 pu for m=1/1 -> Product/2
  Step/1 -> Switch/2
  Current Limit Logic/1(I_ref_sat) -> Current Control/1(i_cv_ref), Vmd13/1
  From17/1 -> RL filter/1(In1)
  omega_ref/1 -> RL filter/5(In5)
  From1/1 -> Current Control/3(i_o)
  Transport Delay1/1 -> RL filter/3(In3)
  Sum2/1 -> Virtual Admittance1/1(delvdq)
  Kip6/1 -> PLL>>grid2/1(vgdq)
  From4/1 -> Current Control/2(v_o)
  From18/1 -> RL filter/4(In4)
  Sum1/1 -> PLL>>grid2/2(thetaPLL)
  First-Order Filter/1 -> Current Limit Logic/1(I_ref_unsat)
  From2/1 -> Sum1/1
  Virtual Admittance1/1(Idqref) -> First-Order Filter/1
  Constant/1 -> Sum1/2
  From5/1 -> Current Control/4(i_cv)
  Switch/1 -> Product/1
  PLL>>grid2/1(vgDQ) -> I_d_error4/1, Demux4/1
  In1/1 -> Sum2/1, Switch/1
  Current Control/1(v_ref_dq) -> Switch/3
  Product/1 -> Kip6/1
  omega_PLL/1 -> Virtual Admittance1/2(omega_PLL)
  In2/1 -> Sum2/2
  Kip9/1 -> ?
  In4/1 -> Kip9/1

== system martins_version_wconv/GFC_WT/VoltageControl ==
  note: analytical
  note: manual tuning
  ref : Inport
  meas : Inport  Port=2
  I filter meas : Inport  Port=3
  Constant : Constant  Value=0
  Demux1 : Demux  Outputs=[vect vect]
  Demux2 : Demux  Outputs=[vect vect]
  Demux3 : Demux  Outputs=[vect vect]
  Gain4 : Gain  Gain=c_f
  Gain5 : Gain  Gain=c_f
  Mux : Mux  Inputs=[vect vect]
  Mux1 : Mux  Inputs=3
  Mux2 : Mux  Inputs=3
  PID Controller : slpidlib/PID Controller  Controller=PI  Form=Parallel  TimeDomain=Continuous-time  UseExternalTs=off  SampleTime=-1  IntegratorMethod=Forward Euler  FilterMethod=Forward Euler  ControllerParametersSource=internal  P=k_vc  I=z  UseKiTs=off  D=0  N=100  UseFilter=on  TunerSelectOption=Transfer Function Based (PID Tuner App)  InitialConditionSource=internal  InitialConditionForIntegrator=0  InitialConditionForFilter=0  DifferentiatorICPrevScaledInput=0  ExternalReset=none  TrackingMode=off  Kt=1  LimitOutput=off  SatLimitsSource=internal  UpperSaturationLimit=2  LowerSaturationLimit=-2  LinearizeAsGain=off  AntiWindupMode=none  Kb=1  LimitIntegrator=off  UpperIntegratorSaturationLimit=inf  LowerIntegratorSaturationLimit=-inf  POutMin=[]  POutMax=[]  IOutMin=[]  IOutMax=[]  DOutMin=[]  DOutMax=[]  NOutMin=[]  NOutMax=[]  SumOutMin=[]  SumOutMax=[]  SaturationOutMin=[]  SaturationOutMax=[]  PParamMin=[]  PParamMax=[]  IParamMin=[]  IParamMax=[]  DParamMin=[]  DParamMax=[]  NParamMin=[]  NParamMax=[]  KbParamMin=[]  KbParamMax=[]  KtParamMin=[]  KtParamMax=[]  KbOutMin=[]  KbOutMax=[]  KtOutMin=[]  KtOutMax=[]  IntegratorOutMin=[]  IntegratorOutMax=[]  FilterOutMin=[]  FilterOutMax=[]  SumI1OutMin=[]  SumI1OutMax=[]  SumI2OutMin=[]  SumI2OutMax=[]  SumI3OutMin=[]  SumI3OutMax=[]  SumI4OutMin=[]  SumI4OutMax=[]  SumDOutMin=[]  SumDOutMax=[]  DifferentiatorOutMin=[]  DifferentiatorOutMax=[]  FilterDiffOutCoefMin=[]  FilterDiffOutCoefMax=[]  ReciprocalOutMin=[]  ReciprocalOutMax=[]  SumDenOutMin=[]  SumDenOutMax=[]  SumNumOutMin=[]  SumNumOutMax=[]  DivideOutMin=[]  DivideOutMax=[]  UdiffTsProdOutMin=[]  UdiffTsProdOutMax=[]  NTsProdOutMin=[]  NTsProdOutMax=[]  UintegralTsProdOutMin=[]  UintegralTsProdOutMax=[]  UngainTsProdOutMin=[]  UngainTsProdOutMax=[]  ClampingZeroOutDataTypeStr=Inherit: Inherit via back propagation  ClampingZeroOutMin=[]  ClampingZeroOutMax=[]  FilterDenConstantOutDataTypeStr=Inherit: Inherit via back propagation  FilterDenConstantOutMin=[]  FilterDenConstantOutMax=[]  PCopyOutDataTypeStr=Inherit: Inherit via back propagation  PCopyOutMin=[]  PCopyOutMax=[]  NCopyOutDataTypeStr=Inherit: Inherit via back propagation  NCopyOutMin=[]  NCopyOutMax=[]  IntegratorContinuousStateAttributes=''  IntegratorStateMustResolveToSignalObject=off  IntegratorRTWStateStorageClass=Auto  FilterContinuousStateAttributes=''  FilterStateMustResolveToSignalObject=off  FilterRTWStateStorageClass=Auto  ParallelPVariant=InternalParameters  IdealPVariant=Disabled  IVariant=InternalParameters  DVariant=Disabled  IntegratorVariant=Continuous  SatVariant=Disabled  AWVariant=Passthrough  PCopyVariant=Disabled  TRVariant=Disabled  FdbkBlocksVariant=Forward  IdealPFdbkVariant=Disabled  SatFdbkVariant=Disabled  DerivativeFilterVariant=Disabled  NVariant=Disabled  NCopyVariant=Disabled_SignalSpec  FilterICVariant=Disabled  IntegratorICVariant=InternalICs  ExternalResetVariant=Disabled  TRSumVariant=Passthrough  SumFdbkVariant=Disabled  SumVariant=Sum_PI  TsampFilterVariant=InternalTs  TsampNgainVariant=Passthrough  TsampIntegralVariant=Disabled_SignalSpec  ExternalSaturationOutDataTypeStr=Inherit: Same as second input
  PID Controller1 : slpidlib/PID Controller  Controller=PI  Form=Ideal  TimeDomain=Continuous-time  UseExternalTs=off  SampleTime=-1  IntegratorMethod=Forward Euler  FilterMethod=Forward Euler  ControllerParametersSource=internal  P=k_vc  I=z  UseKiTs=off  D=0  N=100  UseFilter=on  TunerSelectOption=Transfer Function Based (PID Tuner App)  InitialConditionSource=internal  InitialConditionForIntegrator=1  InitialConditionForFilter=0  DifferentiatorICPrevScaledInput=0  ExternalReset=none  TrackingMode=off  Kt=1  LimitOutput=off  SatLimitsSource=internal  UpperSaturationLimit=2  LowerSaturationLimit=-2  LinearizeAsGain=off  AntiWindupMode=none  Kb=1  LimitIntegrator=off  UpperIntegratorSaturationLimit=inf  LowerIntegratorSaturationLimit=-inf  POutMin=[]  POutMax=[]  IOutMin=[]  IOutMax=[]  DOutMin=[]  DOutMax=[]  NOutMin=[]  NOutMax=[]  SumOutMin=[]  SumOutMax=[]  SaturationOutMin=[]  SaturationOutMax=[]  PParamMin=[]  PParamMax=[]  IParamMin=[]  IParamMax=[]  DParamMin=[]  DParamMax=[]  NParamMin=[]  NParamMax=[]  KbParamMin=[]  KbParamMax=[]  KtParamMin=[]  KtParamMax=[]  KbOutMin=[]  KbOutMax=[]  KtOutMin=[]  KtOutMax=[]  IntegratorOutMin=[]  IntegratorOutMax=[]  FilterOutMin=[]  FilterOutMax=[]  SumI1OutMin=[]  SumI1OutMax=[]  SumI2OutMin=[]  SumI2OutMax=[]  SumI3OutMin=[]  SumI3OutMax=[]  SumI4OutMin=[]  SumI4OutMax=[]  SumDOutMin=[]  SumDOutMax=[]  DifferentiatorOutMin=[]  DifferentiatorOutMax=[]  FilterDiffOutCoefMin=[]  FilterDiffOutCoefMax=[]  ReciprocalOutMin=[]  ReciprocalOutMax=[]  SumDenOutMin=[]  SumDenOutMax=[]  SumNumOutMin=[]  SumNumOutMax=[]  DivideOutMin=[]  DivideOutMax=[]  UdiffTsProdOutMin=[]  UdiffTsProdOutMax=[]  NTsProdOutMin=[]  NTsProdOutMax=[]  UintegralTsProdOutMin=[]  UintegralTsProdOutMax=[]  UngainTsProdOutMin=[]  UngainTsProdOutMax=[]  ClampingZeroOutDataTypeStr=Inherit: Inherit via back propagation  ClampingZeroOutMin=[]  ClampingZeroOutMax=[]  FilterDenConstantOutDataTypeStr=Inherit: Inherit via back propagation  FilterDenConstantOutMin=[]  FilterDenConstantOutMax=[]  PCopyOutDataTypeStr=Inherit: Inherit via back propagation  PCopyOutMin=[]  PCopyOutMax=[]  NCopyOutDataTypeStr=Inherit: Inherit via back propagation  NCopyOutMin=[]  NCopyOutMax=[]  IntegratorContinuousStateAttributes=''  IntegratorStateMustResolveToSignalObject=off  IntegratorRTWStateStorageClass=Auto  FilterContinuousStateAttributes=''  FilterStateMustResolveToSignalObject=off  FilterRTWStateStorageClass=Auto  ParallelPVariant=Passthrough  IdealPVariant=InternalParameters  IVariant=InternalParameters  DVariant=Disabled  IntegratorVariant=Continuous  SatVariant=Disabled  AWVariant=Passthrough  PCopyVariant=Disabled  TRVariant=Disabled  FdbkBlocksVariant=Forward  IdealPFdbkVariant=Disabled  SatFdbkVariant=Disabled  DerivativeFilterVariant=Disabled  NVariant=Disabled  NCopyVariant=Disabled_SignalSpec  FilterICVariant=Disabled  IntegratorICVariant=InternalICs  ExternalResetVariant=Disabled  TRSumVariant=Passthrough  SumFdbkVariant=Disabled  SumVariant=Sum_PI  TsampFilterVariant=InternalTs  TsampNgainVariant=Passthrough  TsampIntegralVariant=Disabled_SignalSpec  ExternalSaturationOutDataTypeStr=Inherit: Same as second input
  PID Controller2 : slpidlib/PID Controller  Controller=PI  Form=Ideal  TimeDomain=Continuous-time  UseExternalTs=off  SampleTime=-1  IntegratorMethod=Forward Euler  FilterMethod=Forward Euler  ControllerParametersSource=internal  P=0.479  I=1/0.007  UseKiTs=off  D=0  N=100  UseFilter=on  TunerSelectOption=Transfer Function Based (PID Tuner App)  InitialConditionSource=internal  InitialConditionForIntegrator=1  InitialConditionForFilter=0  DifferentiatorICPrevScaledInput=0  ExternalReset=none  TrackingMode=off  Kt=1  LimitOutput=off  SatLimitsSource=internal  UpperSaturationLimit=2  LowerSaturationLimit=-2  LinearizeAsGain=off  AntiWindupMode=none  Kb=1  LimitIntegrator=off  UpperIntegratorSaturationLimit=inf  LowerIntegratorSaturationLimit=-inf  POutMin=[]  POutMax=[]  IOutMin=[]  IOutMax=[]  DOutMin=[]  DOutMax=[]  NOutMin=[]  NOutMax=[]  SumOutMin=[]  SumOutMax=[]  SaturationOutMin=[]  SaturationOutMax=[]  PParamMin=[]  PParamMax=[]  IParamMin=[]  IParamMax=[]  DParamMin=[]  DParamMax=[]  NParamMin=[]  NParamMax=[]  KbParamMin=[]  KbParamMax=[]  KtParamMin=[]  KtParamMax=[]  KbOutMin=[]  KbOutMax=[]  KtOutMin=[]  KtOutMax=[]  IntegratorOutMin=[]  IntegratorOutMax=[]  FilterOutMin=[]  FilterOutMax=[]  SumI1OutMin=[]  SumI1OutMax=[]  SumI2OutMin=[]  SumI2OutMax=[]  SumI3OutMin=[]  SumI3OutMax=[]  SumI4OutMin=[]  SumI4OutMax=[]  SumDOutMin=[]  SumDOutMax=[]  DifferentiatorOutMin=[]  DifferentiatorOutMax=[]  FilterDiffOutCoefMin=[]  FilterDiffOutCoefMax=[]  ReciprocalOutMin=[]  ReciprocalOutMax=[]  SumDenOutMin=[]  SumDenOutMax=[]  SumNumOutMin=[]  SumNumOutMax=[]  DivideOutMin=[]  DivideOutMax=[]  UdiffTsProdOutMin=[]  UdiffTsProdOutMax=[]  NTsProdOutMin=[]  NTsProdOutMax=[]  UintegralTsProdOutMin=[]  UintegralTsProdOutMax=[]  UngainTsProdOutMin=[]  UngainTsProdOutMax=[]  ClampingZeroOutDataTypeStr=Inherit: Inherit via back propagation  ClampingZeroOutMin=[]  ClampingZeroOutMax=[]  FilterDenConstantOutDataTypeStr=Inherit: Inherit via back propagation  FilterDenConstantOutMin=[]  FilterDenConstantOutMax=[]  PCopyOutDataTypeStr=Inherit: Inherit via back propagation  PCopyOutMin=[]  PCopyOutMax=[]  NCopyOutDataTypeStr=Inherit: Inherit via back propagation  NCopyOutMin=[]  NCopyOutMax=[]  IntegratorContinuousStateAttributes=''  IntegratorStateMustResolveToSignalObject=off  IntegratorRTWStateStorageClass=Auto  FilterContinuousStateAttributes=''  FilterStateMustResolveToSignalObject=off  FilterRTWStateStorageClass=Auto  ParallelPVariant=Passthrough  IdealPVariant=InternalParameters  IVariant=InternalParameters  DVariant=Disabled  IntegratorVariant=Continuous  SatVariant=Disabled  AWVariant=Passthrough  PCopyVariant=Disabled  TRVariant=Disabled  FdbkBlocksVariant=Forward  IdealPFdbkVariant=Disabled  SatFdbkVariant=Disabled  DerivativeFilterVariant=Disabled  NVariant=Disabled  NCopyVariant=Disabled_SignalSpec  FilterICVariant=Disabled  IntegratorICVariant=InternalICs  ExternalResetVariant=Disabled  TRSumVariant=Passthrough  SumFdbkVariant=Disabled  SumVariant=Sum_PI  TsampFilterVariant=InternalTs  TsampNgainVariant=Passthrough  TsampIntegralVariant=Disabled_SignalSpec  ExternalSaturationOutDataTypeStr=Inherit: Same as second input
  PID Controller3 : slpidlib/PID Controller  Controller=PI  Form=Parallel  TimeDomain=Continuous-time  UseExternalTs=off  SampleTime=-1  IntegratorMethod=Forward Euler  FilterMethod=Forward Euler  ControllerParametersSource=internal  P=0.479  I=1/0.007  UseKiTs=off  D=0  N=100  UseFilter=on  TunerSelectOption=Transfer Function Based (PID Tuner App)  InitialConditionSource=internal  InitialConditionForIntegrator=0  InitialConditionForFilter=0  DifferentiatorICPrevScaledInput=0  ExternalReset=none  TrackingMode=off  Kt=1  LimitOutput=off  SatLimitsSource=internal  UpperSaturationLimit=2  LowerSaturationLimit=-2  LinearizeAsGain=off  AntiWindupMode=none  Kb=1  LimitIntegrator=off  UpperIntegratorSaturationLimit=inf  LowerIntegratorSaturationLimit=-inf  POutMin=[]  POutMax=[]  IOutMin=[]  IOutMax=[]  DOutMin=[]  DOutMax=[]  NOutMin=[]  NOutMax=[]  SumOutMin=[]  SumOutMax=[]  SaturationOutMin=[]  SaturationOutMax=[]  PParamMin=[]  PParamMax=[]  IParamMin=[]  IParamMax=[]  DParamMin=[]  DParamMax=[]  NParamMin=[]  NParamMax=[]  KbParamMin=[]  KbParamMax=[]  KtParamMin=[]  KtParamMax=[]  KbOutMin=[]  KbOutMax=[]  KtOutMin=[]  KtOutMax=[]  IntegratorOutMin=[]  IntegratorOutMax=[]  FilterOutMin=[]  FilterOutMax=[]  SumI1OutMin=[]  SumI1OutMax=[]  SumI2OutMin=[]  SumI2OutMax=[]  SumI3OutMin=[]  SumI3OutMax=[]  SumI4OutMin=[]  SumI4OutMax=[]  SumDOutMin=[]  SumDOutMax=[]  DifferentiatorOutMin=[]  DifferentiatorOutMax=[]  FilterDiffOutCoefMin=[]  FilterDiffOutCoefMax=[]  ReciprocalOutMin=[]  ReciprocalOutMax=[]  SumDenOutMin=[]  SumDenOutMax=[]  SumNumOutMin=[]  SumNumOutMax=[]  DivideOutMin=[]  DivideOutMax=[]  UdiffTsProdOutMin=[]  UdiffTsProdOutMax=[]  NTsProdOutMin=[]  NTsProdOutMax=[]  UintegralTsProdOutMin=[]  UintegralTsProdOutMax=[]  UngainTsProdOutMin=[]  UngainTsProdOutMax=[]  ClampingZeroOutDataTypeStr=Inherit: Inherit via back propagation  ClampingZeroOutMin=[]  ClampingZeroOutMax=[]  FilterDenConstantOutDataTypeStr=Inherit: Inherit via back propagation  FilterDenConstantOutMin=[]  FilterDenConstantOutMax=[]  PCopyOutDataTypeStr=Inherit: Inherit via back propagation  PCopyOutMin=[]  PCopyOutMax=[]  NCopyOutDataTypeStr=Inherit: Inherit via back propagation  NCopyOutMin=[]  NCopyOutMax=[]  IntegratorContinuousStateAttributes=''  IntegratorStateMustResolveToSignalObject=off  IntegratorRTWStateStorageClass=Auto  FilterContinuousStateAttributes=''  FilterStateMustResolveToSignalObject=off  FilterRTWStateStorageClass=Auto  ParallelPVariant=InternalParameters  IdealPVariant=Disabled  IVariant=InternalParameters  DVariant=Disabled  IntegratorVariant=Continuous  SatVariant=Disabled  AWVariant=Passthrough  PCopyVariant=Disabled  TRVariant=Disabled  FdbkBlocksVariant=Forward  IdealPFdbkVariant=Disabled  SatFdbkVariant=Disabled  DerivativeFilterVariant=Disabled  NVariant=Disabled  NCopyVariant=Disabled_SignalSpec  FilterICVariant=Disabled  IntegratorICVariant=InternalICs  ExternalResetVariant=Disabled  TRSumVariant=Passthrough  SumFdbkVariant=Disabled  SumVariant=Sum_PI  TsampFilterVariant=InternalTs  TsampNgainVariant=Passthrough  TsampIntegralVariant=Disabled_SignalSpec  ExternalSaturationOutDataTypeStr=Inherit: Same as second input
  Sum1 : Sum  Inputs=|+-
  Sum2 : Sum  Inputs=+-|
  Sum4 : Sum  Inputs=++-
  Sum5 : Sum  Inputs=+++
  Transfer Fcn2 : TransferFcn  Denominator=[0.005 1]
  Transfer Fcn3 : TransferFcn  Denominator=[0.005 1]
  d-axis v control : Scope  NumInputPorts=3
  q-axis v control : Scope  NumInputPorts=3
  I_ref_unsat : Outport
  wires:
  Mux2/1 -> d-axis v control/2
  Transfer Fcn2/1 -> Sum5/3, Mux1/1
  ? -> ?
  PID Controller2/1 -> Mux2/2, Sum4/2
  Mux1/1 -> q-axis v control/2
  Demux3/2 -> Sum2/1
  meas/1 -> Demux1/1
  Gain5/1 -> Mux1/3, Sum5/1
  PID Controller3/1 -> Sum5/2, Mux1/2
  Demux2/2 -> Transfer Fcn2/1
  Sum5/1 -> Mux/2, q-axis v control/3
  Mux/1 -> I_ref_unsat/1
  Gain4/1 -> Mux2/3, Sum4/3
  Demux1/2 -> Gain4/1, Sum2/2
  Sum1/1 -> PID Controller2/1, d-axis v control/1
  Demux1/1 -> Sum1/2, Gain5/1
  ref/1 -> Demux3/1
  Sum2/1 -> PID Controller3/1, q-axis v control/1
  Transfer Fcn3/1 -> Mux2/1, Sum4/1
  Demux2/1 -> Transfer Fcn3/1
  I filter meas/1 -> Demux2/1
  Sum4/1 -> Mux/1, d-axis v control/3
  Demux3/1 -> Sum1/1

== system martins_version_wconv/GFC_WT/grid>>PLL1 ==
  note: [  al
      |     be  ]
  note: [ d
      |    q ]
  note: [  cos(wt)   -sin(wt)
      |    sin(wt)    cos(wt)   ]
  note: =
  note: *
  note: [  al
      |     be  ]
  note: [ d
      |    q ]
  note: inv ([  cos(wt)   sin(wt)
      |    -sin(wt)    cos(wt)   ])
  note: =
  note: *
  vgDQ : Inport
  wt : Inport  Port=2
  Cos : Trigonometry  Operator=cos
  Demux1 : Demux  Outputs=[vect vect]
  Display5 : Display
  Mux3 : Mux  Inputs=2
  Product{,1..3} (4 alike) : Product
  Sin : Trigonometry
  Sum : Sum
  Sum1 : Sum  Inputs=+-
  vgdq : Outport  InitialOutput=[0,0]  VectorParamsAs1DForOutWhenUnconnected=off
  wires:
  Product3/1 -> Sum1/2
  Demux1/2 -> Product2/1, Product1/1
  Product2/1 -> Sum1/1
  Cos/1 -> Product2/2, Product/2
  Product1/1 -> Sum/2
  Sin/1 -> Product3/2, Product1/2
  vgDQ/1 -> Demux1/1
  Sum1/1 -> Mux3/2
  Mux3/1 -> vgdq/1, Display5/1
  Sum/1 -> Mux3/1
  Product/1 -> Sum/1
  wt/1 -> Cos/1, Sin/1
  Demux1/1 -> Product3/1, Product/1
